simulink model "Robot"  (R2018a)
settings: Solver=VariableStepAuto  StartTime=0.0  StopTime=inf  FixedStep=1e-4  RelTol=1e-3  EnableMultiTasking=on
values from neighbouring files (symbols this model uses):
  CM730_acc_center = (4 * 9.80665)    (= 39.2266)    [CM730.m]
  CM730_acc_gain = 512 / CM730_acc_center    (= 13.0523675261)    [CM730.m]
  CM730_gyro_center = (1600 / 360 * 2 * pi)    (= 27.9252680319)    [CM730.m]
  CM730_gyro_gain = 512 / CM730_gyro_center    (= 18.3346494442)    [CM730.m]
  CM730_sample_time = 1e-3    (= 0.001)    [CM730.m]
  FSR_max = 254    [FSR.m]
  FSR_no_load = 255    [FSR.m]
  FSR_sample_time = 0.001    [FSR.m]
  FSR_scale = 1000    [FSR.m]
  g = 0    [Euler.m]
  MX106_Te = 1/1000    (= 0.001)    [MX106_init.m]
  MX28_inertia = 9e-8 * MX28_reduction^2    (= 0.0033385284)    [MX28_init.m]
  MX28_Te = 1/1000    (= 0.001)    [MX28_init.m]
  posZero_ID1 = posZero(1)    [Robot_init.m]
  posZero_ID10 = posZero(14)    [Robot_init.m]
  posZero_ID11 = posZero(9)    [Robot_init.m]
  posZero_ID12 = posZero(15)    [Robot_init.m]
  posZero_ID13 = posZero(10)    [Robot_init.m]
  posZero_ID14 = posZero(16)    [Robot_init.m]
  posZero_ID15 = posZero(11)    [Robot_init.m]
  posZero_ID16 = posZero(17)    [Robot_init.m]
  posZero_ID17 = posZero(12)    [Robot_init.m]
  posZero_ID18 = posZero(18)    [Robot_init.m]
  posZero_ID19 = posZero(19)    [Robot_init.m]
  posZero_ID2 = posZero(4)    [Robot_init.m]
  posZero_ID20 = posZero(20)    [Robot_init.m]
  posZero_ID3 = posZero(2)    [Robot_init.m]
  posZero_ID4 = posZero(5)    [Robot_init.m]
  posZero_ID5 = posZero(3)    [Robot_init.m]
  posZero_ID6 = posZero(6)    [Robot_init.m]
  posZero_ID7 = posZero(7)    [Robot_init.m]
  posZero_ID8 = posZero(13)    [Robot_init.m]
  posZero_ID9 = posZero(8)    [Robot_init.m]
  robot_chest_mass = 2385.0    (= 2385)    [Robot_init.m]
  robot_floor_friction_coeff = 0.6    [Robot_init.m]
  robot_floor_position_gain = -1e5    (= -100000)    [Robot_init.m]
  robot_floor_speed_gain = -1e3    (= -1000)    [Robot_init.m]
  robot_gravity = [0 0 0]    [Robot_init.m]
  robot_head_mass = 177.69    [Robot_init.m]
  robot_hip1_mass = 49.00    (= 49)    [Robot_init.m]
  robot_left_ankle_mass = 360.00    (= 360)    [Robot_init.m]
  robot_left_foot_mass = 267.00    (= 267)    [Robot_init.m]
  robot_left_forearm_mass = 248.00    (= 248)    [Robot_init.m]
  robot_left_hip2_mass = 358.00    (= 358)    [Robot_init.m]
  robot_left_lower_leg_mass = 129.00    (= 129)    [Robot_init.m]
  robot_left_shoulder_mass = 39.00    (= 39)    [Robot_init.m]
  robot_left_thigh_mass = 1263.00    (= 1263)    [Robot_init.m]
  robot_left_upper_arm_mass = 247.00    (= 247)    [Robot_init.m]
  robot_neck_mass = 90    [Robot_init.m]
  robot_right_ankle_mass = 360.00    (= 360)    [Robot_init.m]
  robot_right_foot_mass = 267.00    (= 267)    [Robot_init.m]
  robot_right_forearm_mass = 248.00    (= 248)    [Robot_init.m]
  robot_right_hip2_mass = 358.00    (= 358)    [Robot_init.m]
  robot_right_lower_leg_mass = 129.00    (= 129)    [Robot_init.m]
  robot_right_shoulder_mass = 39.00    (= 39)    [Robot_init.m]
  robot_right_thigh_mass = 263.00    (= 263)    [Robot_init.m]
  robot_right_upper_arm_mass = 247.00    (= 247)    [Robot_init.m]
  X = get(hObject,'Value')    [gui_kine.m]
  Y = get(hObject,'Value')    [gui_kine.m]
  Z = get(hObject,'Value')    [gui_kine.m]
libraries: sm_lib x167, fl_lib x128, nesl_utility x77, dspindex x1
(part 5 of 7)

== system Robot/Robot simulation/Right Arm/Right Shoulder Roll (3) ==
  Inertia : sm_lib/Body Elements/Inertia  InertiaType=Custom  Mass=1  MassUnits=g  CenterOfMass=[0 0 0]  CenterOfMassUnits=m  MomentsOfInertia=[0 0 MX28_inertia]  MomentsOfInertiaUnits=kg*m^2  ProductsOfInertia=[0 0 0]  ProductsOfInertiaUnits=kg*m^2  GraphicType=Marker  MarkerShape=Inertia  MarkerSize=20  GraphicVisPropType=SimpleVisualProperties  GraphicDiffuseColor=[0.5 0.5 0.5]  GraphicSpecularColor=[0.5 0.5 0.5 1.0]  GraphicAmbientColor=[0.15 0.15 0.15 1.0]  GraphicEmissiveColor=[0.0 0.0 0.0 1.0]  GraphicShininess=75  GraphicOpacity=1.0
  MX28 Command : DataStoreRead  DataStoreName=MX28_ID3  SampleTime=MX28_Te  DataStoreElements=MX28_ID3.CW_angle_limit#MX28_ID3.CCW_angle_limit#MX28_ID3.torque_enable#MX28_ID3.D_gain#MX28_ID3.I_gain#MX28_ID3.P_gain#MX28_ID3.goal_position#MX28_ID3.moving_speed#MX28_ID3.torque_limit
  MX28 State : DataStoreWrite  DataStoreName=MX28_ID3  DataStoreElements=MX28_ID3.present_position#MX28_ID3.present_speed#MX28_ID3.present_load#MX28_ID3.moving#MX28_ID3.pwm
  Model : ModelReference  ModelNameDialog=MX28.slx  SimulationMode=Normal  ModelReferenceVersion=1.66
  Position converter : nesl_utility/PS-Simulink Converter  PhysicalDomain=network_engine_domain  SubClassName=ps_output  LeftPortType=input  RightPortType=output  PseudoPeriodic=off  Frequencies=[]  Unit=rad  AffineConversion=off
  Revolute Joint : sm_lib/Joints/Revolute Joint  SenseConstraintForce=off  SenseConstraintForceX=off  SenseConstraintForceY=off  SenseConstraintForceZ=off  SenseConstraintTorque=off  SenseConstraintTorqueX=off  SenseConstraintTorqueY=off  SenseConstraintTorqueZ=off  SenseTotalForce=off  SenseTotalForceX=off  SenseTotalForceY=off  SenseTotalForceZ=off  SenseTotalTorque=off  SenseTotalTorqueX=off  SenseTotalTorqueY=off  SenseTotalTorqueZ=off  CompositeWrenchDir=FollowerOnBase  CompositeWrenchFrame=BaseFrame  EquilibriumPosition=0  EquilibriumPositionUnits=deg  SpringStiffness=0  SpringStiffnessUnits=N*m/deg  DampingCoefficient=MX28_lub_friction  DampingCoefficientUnits=N*m/(rad/s)  TorqueActuationMode=InputTorque  MotionActuationMode=ComputedMotion  SensePosition=on  SenseVelocity=on  SenseAcceleration=off  SenseTorqueForce=off  PositionTargetSpecify=on  PositionTargetPriority=High  PositionTargetValue=MX28_init_position  PositionTargetValueUnits=rad  VelocityTargetSpecify=on  VelocityTargetPriority=High  VelocityTargetValue=MX28_init_speed  VelocityTargetValueUnits=rad/s
  Speed converter : nesl_utility/PS-Simulink Converter  PhysicalDomain=network_engine_domain  SubClassName=ps_output  LeftPortType=input  RightPortType=output  PseudoPeriodic=off  Frequencies=[]  Unit=rad/s  AffineConversion=off
  Torque converter : nesl_utility/Simulink-PS Converter  PhysicalDomain=network_engine_domain  SubClassName=ps_input  LeftPortType=input  RightPortType=output  PseudoPeriodic=off  Frequencies=[]  NoiseDistribution=none  NoiseParameters=[]  Unit=N*m  AffineConversion=off  FilteringAndDerivatives=zero  SimscapeFilterOrder=1  InputFilterTimeConstant=0.001  UdotUserProvided=1
  Base : PMIOPort  Side=Left
  Axis : PMIOPort  Port=2  Side=Right
  wires:
  Model/4 -> MX28 State/3
  Model/2 -> MX28 State/1
  Model/5 -> MX28 State/4
  Model/3 -> MX28 State/2
  MX28 Command/3 -> Model/5
  MX28 Command/6 -> Model/8
  MX28 Command/4 -> Model/6
  MX28 Command/5 -> Model/7
  MX28 Command/7 -> Model/9
  MX28 Command/2 -> Model/4
  MX28 Command/1 -> Model/3
  Speed converter/1 -> Model/1
  Position converter/1 -> Model/2
  Model/1 -> Torque converter/1
  Model/6 -> MX28 State/5
  MX28 Command/8 -> Model/10
  MX28 Command/9 -> Model/11
  connections:
  Axis/RConn1 -- Revolute Joint/RConn1 -- Inertia/RConn1
  Revolute Joint/RConn3 -- Speed converter/LConn1
  Revolute Joint/RConn2 -- Position converter/LConn1
  Revolute Joint/LConn2 -- Torque converter/RConn1
  Revolute Joint/LConn1 -- Base/RConn1

== system Robot/Robot simulation/Right Arm/Right Upper Arm ==
  Right Arm Axis to Right Forearm Base : sm_lib/Frames and Transforms/Rigid Transform  TranslationMethod=Cartesian  TranslationStandardOffset=0  TranslationLengthUnit=mm  TranslationStandardAxis=+Z  TranslationCartesianOffset=robot_right_upper_arm_to_right_forearm_tra  TranslationROffset=0  TranslationROffsetUnits=m  TranslationZOffset=0  TranslationZOffsetUnits=m  TranslationThetaOffset=0  TranslationThetaOffsetUnits=deg  RotationMethod=RotationMatrix  RotationAngleUnits=deg  RotationStandardAxis=+Z  RotationAngle=0  RotationArbitraryAxis=[0 0 1]  FollAlignAxisA=+X  BaseAlignAxisA=-Y  FollAlignAxisB=+Z  BaseAlignAxisB=+X  RotationSequenceAxes=FollowerAxes  RotationSequence=XYX  RotationSequenceAngles=[0 0 0]  RotationSequenceAnglesUnits=deg  RotationMatrix=robot_right_upper_arm_to_right_forearm_rot
  Solid : sm_lib/Body Elements/Solid  InertiaType=Custom  Mass=robot_right_upper_arm_mass  MassUnits=g  CenterOfMass=robot_right_upper_arm_to_center_mass  CenterOfMassUnits=mm  MomentsOfInertia=robot_right_upper_arm_moment_inertia  MomentsOfInertiaUnits=g*mm^2  ProductsOfInertia=robot_right_upper_arm_product_inertia  ProductsOfInertiaUnits=g*mm^2  DensityBased=on  Density=1000  DensityUnits=kg/(m^3)  DoExposeReferenceFrame=on  SerializedFrames=<Frames/>  GraphicType=FromGeometry  MarkerShape=Sphere  MarkerSize=10  MarkerSizeUnits=m  GraphicVisPropType=SimpleVisualProperties  GraphicDiffuseColor=[0.5 0.5 0.5]  GraphicSpecularColor=[0.5 0.5 0.5 1.0]  GraphicAmbientColor=[0.15 0.15 0.15 1.0]  GraphicEmissiveColor=[0.0 0.0 0.0 1.0]  GraphicShininess=75  GraphicOpacity=1.0  GeometryShape=FromFile  RectangleSize=[1 1]  RectangleSizeUnits=m  BrickDimensions=[1 1 1]  BrickDimensionUnits=mm  CylinderRadius=1  CylinderRadiusUnits=m  CylinderLength=1  CylinderLengthUnits=m  SphereRadius=1  SphereRadiusUnits=m  EllipsoidRadii=[1 1 1]  EllipsoidRadiiUnits=m  ExtrusionCrossSection=[1 1; -1 1; -1 -1; 1 -1]  ExtrusionCrossSectionUnits=m  ExtrusionLength=1  ExtrusionLengthUnits=m  PolygonNumSides=3  PolygonOuterRadius=1  PolygonOuterRadiusUnits=m  ExtGeomFileType=STL  ExtGeomFileName=\STL\Right_Arm.STL  ExtGeomFileUnits=mm  RevolutionCrossSection=[1 1; 1 -1; 2 -1; 2 1]  RevolutionCrossSectionUnits=m  RevolutionExtent=Full  RevolutionAngle=180  RevolutionAngleUnits=deg
  Right Shoulder Roll : PMIOPort  Side=Left
  Right Elbow : PMIOPort  Port=2  Side=Right
  connections:
  Right Arm Axis to Right Forearm Base/LConn1 -- Right Shoulder Roll/RConn1 -- Solid/RConn1
  Right Arm Axis to Right Forearm Base/RConn1 -- Right Elbow/RConn1

== system Robot/Robot simulation/Right Leg/Floor model ==
  note: Left foot:
      | 1 = back right
      | 2 = back left
      | 3 = front left
      | 4 = front right
  note: Right foot:
      | 1 = front left
      | 2 = front right
      | 3 = back right
      | 4 = back left
  Back Left Scale : Gain  Gain=FSR_scale  OutDataTypeStr=uint16  SampleTime=FSR_sample_time  SaturateOnIntegerOverflow=on
  Back Right Scale : Gain  Gain=FSR_scale  OutDataTypeStr=uint16  SampleTime=FSR_sample_time  SaturateOnIntegerOverflow=on
  Data Store Write : DataStoreWrite  DataStoreName=FSR_ID111  DataStoreElements=FSR_ID111.fsr_1#FSR_ID111.fsr_2#FSR_ID111.fsr_3#FSR_ID111.fsr_4#FSR_ID111.fsr_x#FSR_ID111.fsr_y
  Divide X : Product  Inputs=*/
  Divide Y : Product  Inputs=*/
  Floor Model Back Left : Subsystem
  Floor Model Back Right : Subsystem
  Floor Model Front Left : Subsystem
  Floor Model Front Right : Subsystem
  Front Left Scale : Gain  Gain=FSR_scale  OutDataTypeStr=uint16  SampleTime=FSR_sample_time  SaturateOnIntegerOverflow=on
  Front Right Scale : Gain  Gain=FSR_scale  OutDataTypeStr=uint16  SampleTime=FSR_sample_time  SaturateOnIntegerOverflow=on
  Gain X : Gain  Gain=FSR_max  OutDataTypeStr=uint8  SaturateOnIntegerOverflow=on
  Gain Y : Gain  Gain=FSR_max  OutDataTypeStr=uint8  SaturateOnIntegerOverflow=on
  No load : Constant  Value=FSR_no_load  OutDataTypeStr=uint8
  Switch X : Switch  Criteria=u2 > Threshold
  Switch Y : Switch  Criteria=u2 > Threshold
  Total : Sum  Inputs=++++  SampleTime=FSR_sample_time
  Total Back : Sum  SampleTime=FSR_sample_time
  Total Right : Sum  SampleTime=FSR_sample_time
  Front Left : PMIOPort  Side=Left
  Front Right : PMIOPort  Port=2  Side=Left
  Back Right : PMIOPort  Port=3  Side=Left
  Back Left : PMIOPort  Port=4  Side=Left
  Floor : PMIOPort  Port=5  Side=Right
  wires:
  Floor Model Front Left/1(Z force) -> Total/1, Front Left Scale/1
  Floor Model Front Right/1(Z force) -> Total Right/1, Front Right Scale/1, Total/2
  Floor Model Back Right/1(Z force) -> Total Back/1, Total/3, Back Right Scale/1, Total Right/2
  Floor Model Back Left/1(Z force) -> Total Back/2, Total/4, Back Left Scale/1
  Total/1 -> Divide Y/2, Divide X/2, Switch Y/2, Switch X/2
  No load/1 -> Switch Y/3, Switch X/3
  Divide X/1 -> Gain X/1
  Total Right/1 -> Divide X/1
  Divide Y/1 -> Gain Y/1
  Total Back/1 -> Divide Y/1
  Gain X/1 -> Switch X/1
  Gain Y/1 -> Switch Y/1
  Switch X/1 -> Data Store Write/5
  Switch Y/1 -> Data Store Write/6
  Front Left Scale/1 -> Data Store Write/1
  Front Right Scale/1 -> Data Store Write/2
  Back Right Scale/1 -> Data Store Write/3
  Back Left Scale/1 -> Data Store Write/4
  connections:
  Floor Model Back Left/LConn1 -- Back Left/RConn1
  Floor Model Back Right/LConn1 -- Back Right/RConn1
  Floor Model Front Right/LConn1 -- Front Right/RConn1
  Floor Model Front Left/LConn1 -- Front Left/RConn1
  Floor/RConn1 -- Floor Model Front Left/RConn1 -- Floor Model Front Right/RConn1 -- Floor Model Back Right/RConn1 -- Floor Model Back Left/RConn1

== system Robot/Robot simulation/Right Leg/Right Ankle ==
  Right Ankle Base to Right Foot Base : sm_lib/Frames and Transforms/Rigid Transform  TranslationMethod=Cartesian  TranslationStandardOffset=0  TranslationLengthUnit=mm  TranslationStandardAxis=+Z  TranslationCartesianOffset=robot_right_ankle_to_right_foot_tra  TranslationROffset=0  TranslationROffsetUnits=m  TranslationZOffset=0  TranslationZOffsetUnits=m  TranslationThetaOffset=0  TranslationThetaOffsetUnits=deg  RotationMethod=RotationMatrix  RotationAngleUnits=deg  RotationStandardAxis=+Z  RotationAngle=0  RotationArbitraryAxis=[0 0 1]  FollAlignAxisA=+X  BaseAlignAxisA=+Z  FollAlignAxisB=+Y  BaseAlignAxisB=-Y  RotationSequenceAxes=FollowerAxes  RotationSequence=XYX  RotationSequenceAngles=[0 0 0]  RotationSequenceAnglesUnits=deg  RotationMatrix=robot_right_ankle_to_right_foot_rot
  Solid : sm_lib/Body Elements/Solid  InertiaType=Custom  Mass=robot_right_ankle_mass  MassUnits=g  CenterOfMass=robot_right_ankle_to_center_mass  CenterOfMassUnits=mm  MomentsOfInertia=robot_right_ankle_moment_inertia  MomentsOfInertiaUnits=g*mm^2  ProductsOfInertia=robot_right_ankle_product_inertia  ProductsOfInertiaUnits=g*mm^2  DensityBased=on  Density=1000  DensityUnits=kg/(m^3)  DoExposeReferenceFrame=on  SerializedFrames=<Frames/>  GraphicType=FromGeometry  MarkerShape=Sphere  MarkerSize=10  MarkerSizeUnits=m  GraphicVisPropType=SimpleVisualProperties  GraphicDiffuseColor=[0.5 0.5 0.5]  GraphicSpecularColor=[0.5 0.5 0.5 1.0]  GraphicAmbientColor=[0.15 0.15 0.15 1.0]  GraphicEmissiveColor=[0.0 0.0 0.0 1.0]  GraphicShininess=75  GraphicOpacity=1.0  GeometryShape=FromFile  RectangleSize=[1 1]  RectangleSizeUnits=m  BrickDimensions=[1 1 1]  BrickDimensionUnits=m  CylinderRadius=1  CylinderRadiusUnits=m  CylinderLength=1  CylinderLengthUnits=m  SphereRadius=1  SphereRadiusUnits=m  EllipsoidRadii=[1 1 1]  EllipsoidRadiiUnits=m  ExtrusionCrossSection=[1 1; -1 1; -1 -1; 1 -1]  ExtrusionCrossSectionUnits=m  ExtrusionLength=1  ExtrusionLengthUnits=m  PolygonNumSides=3  PolygonOuterRadius=1  PolygonOuterRadiusUnits=m  ExtGeomFileType=STL  ExtGeomFileName=\STL\Right_Ankle.STL  ExtGeomFileUnits=mm  RevolutionCrossSection=[1 1; 1 -1; 2 -1; 2 1]  RevolutionCrossSectionUnits=m  RevolutionExtent=Full  RevolutionAngle=180  RevolutionAngleUnits=deg
  Right Ankle Pitch : PMIOPort  Side=Left
  Right Ankle Roll : PMIOPort  Port=2  Side=Right
  connections:
  Solid/RConn1 -- Right Ankle Base to Right Foot Base/LConn1 -- Right Ankle Pitch/RConn1
  Right Ankle Roll/RConn1 -- Right Ankle Base to Right Foot Base/RConn1

== system Robot/Robot simulation/Right Leg/Right Ankle Pitch (15) ==
  Inertia : sm_lib/Body Elements/Inertia  InertiaType=Custom  Mass=1  MassUnits=g  CenterOfMass=[0 0 0]  CenterOfMassUnits=m  MomentsOfInertia=[0 0 MX28_inertia]  MomentsOfInertiaUnits=kg*m^2  ProductsOfInertia=[0 0 0]  ProductsOfInertiaUnits=kg*m^2  GraphicType=Marker  MarkerShape=Inertia  MarkerSize=20  GraphicVisPropType=SimpleVisualProperties  GraphicDiffuseColor=[0.5 0.5 0.5]  GraphicSpecularColor=[0.5 0.5 0.5 1.0]  GraphicAmbientColor=[0.15 0.15 0.15 1.0]  GraphicEmissiveColor=[0.0 0.0 0.0 1.0]  GraphicShininess=75  GraphicOpacity=1.0
  MX106 Command : DataStoreRead  DataStoreName=MX106_ID15  SampleTime=MX106_Te  DataStoreElements=MX106_ID15.CW_angle_limit#MX106_ID15.CCW_angle_limit#MX106_ID15.torque_enable#MX106_ID15.D_gain#MX106_ID15.I_gain#MX106_ID15.P_gain#MX106_ID15.goal_position#MX106_ID15.moving_speed#MX106_ID15.torque_limit
  MX106 State : DataStoreWrite  DataStoreName=MX106_ID15  DataStoreElements=MX106_ID15.present_position#MX106_ID15.present_speed#MX106_ID15.present_load#MX106_ID15.moving#MX106_ID15.pwm
  Model : ModelReference  ModelNameDialog=MX106.slx  SimulationMode=Normal  ModelReferenceVersion=1.67
  Position converter : nesl_utility/PS-Simulink Converter  PhysicalDomain=network_engine_domain  SubClassName=ps_output  LeftPortType=input  RightPortType=output  PseudoPeriodic=off  Frequencies=[]  Unit=rad  AffineConversion=off
  Revolute Joint : sm_lib/Joints/Revolute Joint  SenseConstraintForce=off  SenseConstraintForceX=off  SenseConstraintForceY=off  SenseConstraintForceZ=off  SenseConstraintTorque=off  SenseConstraintTorqueX=off  SenseConstraintTorqueY=off  SenseConstraintTorqueZ=off  SenseTotalForce=off  SenseTotalForceX=off  SenseTotalForceY=off  SenseTotalForceZ=off  SenseTotalTorque=off  SenseTotalTorqueX=off  SenseTotalTorqueY=off  SenseTotalTorqueZ=off  CompositeWrenchDir=FollowerOnBase  CompositeWrenchFrame=BaseFrame  EquilibriumPosition=0  EquilibriumPositionUnits=deg  SpringStiffness=0  SpringStiffnessUnits=N*m/deg  DampingCoefficient=MX28_lub_friction  DampingCoefficientUnits=N*m/(rad/s)  TorqueActuationMode=InputTorque  MotionActuationMode=ComputedMotion  SensePosition=on  SenseVelocity=on  SenseAcceleration=off  SenseTorqueForce=off  PositionTargetSpecify=on  PositionTargetPriority=High  PositionTargetValue=MX28_init_position  PositionTargetValueUnits=rad  VelocityTargetSpecify=on  VelocityTargetPriority=High  VelocityTargetValue=MX28_init_speed  VelocityTargetValueUnits=rad/s
  Speed converter : nesl_utility/PS-Simulink Converter  PhysicalDomain=network_engine_domain  SubClassName=ps_output  LeftPortType=input  RightPortType=output  PseudoPeriodic=off  Frequencies=[]  Unit=rad/s  AffineConversion=off
  Torque converter : nesl_utility/Simulink-PS Converter  PhysicalDomain=network_engine_domain  SubClassName=ps_input  LeftPortType=input  RightPortType=output  PseudoPeriodic=off  Frequencies=[]  NoiseDistribution=none  NoiseParameters=[]  Unit=N*m  AffineConversion=off  FilteringAndDerivatives=zero  SimscapeFilterOrder=1  InputFilterTimeConstant=0.001  UdotUserProvided=1
  Base : PMIOPort  Side=Left
  Axis : PMIOPort  Port=2  Side=Right
  wires:
  Model/4 -> MX106 State/3
  Model/2 -> MX106 State/1
  Model/5 -> MX106 State/4
  Model/3 -> MX106 State/2
  MX106 Command/3 -> Model/5
  MX106 Command/6 -> Model/8
  MX106 Command/4 -> Model/6
  MX106 Command/5 -> Model/7
  MX106 Command/7 -> Model/9
  MX106 Command/2 -> Model/4
  MX106 Command/1 -> Model/3
  Position converter/1 -> Model/2
  Speed converter/1 -> Model/1
  Model/1 -> Torque converter/1
  Model/6 -> MX106 State/5
  MX106 Command/8 -> Model/10
  MX106 Command/9 -> Model/11
  connections:
  Axis/RConn1 -- Revolute Joint/RConn1 -- Inertia/RConn1
  Revolute Joint/LConn1 -- Base/RConn1
  Revolute Joint/RConn3 -- Speed converter/LConn1
  Revolute Joint/RConn2 -- Position converter/LConn1
  Revolute Joint/LConn2 -- Torque converter/RConn1

== system Robot/Robot simulation/Right Leg/Right Ankle Roll (17) ==
  Inertia : sm_lib/Body Elements/Inertia  InertiaType=Custom  Mass=1  MassUnits=g  CenterOfMass=[0 0 0]  CenterOfMassUnits=m  MomentsOfInertia=[0 0 MX28_inertia]  MomentsOfInertiaUnits=kg*m^2  ProductsOfInertia=[0 0 0]  ProductsOfInertiaUnits=kg*m^2  GraphicType=Marker  MarkerShape=Inertia  MarkerSize=20  GraphicVisPropType=SimpleVisualProperties  GraphicDiffuseColor=[0.5 0.5 0.5]  GraphicSpecularColor=[0.5 0.5 0.5 1.0]  GraphicAmbientColor=[0.15 0.15 0.15 1.0]  GraphicEmissiveColor=[0.0 0.0 0.0 1.0]  GraphicShininess=75  GraphicOpacity=1.0
  MX106 Command : DataStoreRead  DataStoreName=MX106_ID17  SampleTime=MX106_Te  DataStoreElements=MX106_ID17.CW_angle_limit#MX106_ID17.CCW_angle_limit#MX106_ID17.torque_enable#MX106_ID17.D_gain#MX106_ID17.I_gain#MX106_ID17.P_gain#MX106_ID17.goal_position#MX106_ID17.moving_speed#MX106_ID17.torque_limit
  MX106 State : DataStoreWrite  DataStoreName=MX106_ID17  DataStoreElements=MX106_ID17.present_position#MX106_ID17.present_speed#MX106_ID17.present_load#MX106_ID17.moving#MX106_ID17.pwm
  Model : ModelReference  ModelNameDialog=MX106.slx  SimulationMode=Normal  ModelReferenceVersion=1.67
  Position converter : nesl_utility/PS-Simulink Converter  PhysicalDomain=network_engine_domain  SubClassName=ps_output  LeftPortType=input  RightPortType=output  PseudoPeriodic=off  Frequencies=[]  Unit=rad  AffineConversion=off
  Revolute Joint : sm_lib/Joints/Revolute Joint  SenseConstraintForce=off  SenseConstraintForceX=off  SenseConstraintForceY=off  SenseConstraintForceZ=off  SenseConstraintTorque=off  SenseConstraintTorqueX=off  SenseConstraintTorqueY=off  SenseConstraintTorqueZ=off  SenseTotalForce=off  SenseTotalForceX=off  SenseTotalForceY=off  SenseTotalForceZ=off  SenseTotalTorque=off  SenseTotalTorqueX=off  SenseTotalTorqueY=off  SenseTotalTorqueZ=off  CompositeWrenchDir=FollowerOnBase  CompositeWrenchFrame=BaseFrame  EquilibriumPosition=0  EquilibriumPositionUnits=deg  SpringStiffness=0  SpringStiffnessUnits=N*m/deg  DampingCoefficient=MX28_lub_friction  DampingCoefficientUnits=N*m/(rad/s)  TorqueActuationMode=InputTorque  MotionActuationMode=ComputedMotion  SensePosition=on  SenseVelocity=on  SenseAcceleration=off  SenseTorqueForce=off  PositionTargetSpecify=on  PositionTargetPriority=High  PositionTargetValue=MX28_init_position  PositionTargetValueUnits=rad  VelocityTargetSpecify=on  VelocityTargetPriority=High  VelocityTargetValue=MX28_init_speed  VelocityTargetValueUnits=rad/s
  Speed converter : nesl_utility/PS-Simulink Converter  PhysicalDomain=network_engine_domain  SubClassName=ps_output  LeftPortType=input  RightPortType=output  PseudoPeriodic=off  Frequencies=[]  Unit=rad/s  AffineConversion=off
  Torque converter : nesl_utility/Simulink-PS Converter  PhysicalDomain=network_engine_domain  SubClassName=ps_input  LeftPortType=input  RightPortType=output  PseudoPeriodic=off  Frequencies=[]  NoiseDistribution=none  NoiseParameters=[]  Unit=N*m  AffineConversion=off  FilteringAndDerivatives=zero  SimscapeFilterOrder=1  InputFilterTimeConstant=0.001  UdotUserProvided=1
  Base : PMIOPort  Side=Left
  Axis : PMIOPort  Port=2  Side=Right
  wires:
  Model/4 -> MX106 State/3
  Model/2 -> MX106 State/1
  Model/5 -> MX106 State/4
  Model/3 -> MX106 State/2
  MX106 Command/3 -> Model/5
  MX106 Command/6 -> Model/8
  MX106 Command/4 -> Model/6
  MX106 Command/5 -> Model/7
  MX106 Command/7 -> Model/9
  MX106 Command/2 -> Model/4
  MX106 Command/1 -> Model/3
  Position converter/1 -> Model/2
  Speed converter/1 -> Model/1
  Model/1 -> Torque converter/1
  Model/6 -> MX106 State/5
  MX106 Command/8 -> Model/10
  MX106 Command/9 -> Model/11
  connections:
  Axis/RConn1 -- Revolute Joint/RConn1 -- Inertia/RConn1
  Revolute Joint/LConn1 -- Base/RConn1
  Revolute Joint/RConn3 -- Speed converter/LConn1
  Revolute Joint/RConn2 -- Position converter/LConn1
  Revolute Joint/LConn2 -- Torque converter/RConn1

== system Robot/Robot simulation/Right Leg/Right Foot ==
  Right Foot Axis to Back Left : sm_lib/Frames and Transforms/Rigid Transform  TranslationMethod=Cartesian  TranslationStandardOffset=0  TranslationLengthUnit=mm  TranslationStandardAxis=+Z  TranslationCartesianOffset=robot_right_foot_to_back_left_floor_tra  TranslationROffset=0  TranslationROffsetUnits=m  TranslationZOffset=0  TranslationZOffsetUnits=m  TranslationThetaOffset=0  TranslationThetaOffsetUnits=deg  RotationMethod=RotationMatrix  RotationAngleUnits=deg  RotationStandardAxis=+Z  RotationAngle=0.0  RotationArbitraryAxis=[0 0 1]  FollAlignAxisA=+X  BaseAlignAxisA=-X  FollAlignAxisB=+Z  BaseAlignAxisB=-Y  RotationSequenceAxes=FollowerAxes  RotationSequence=XYX  RotationSequenceAngles=[0 0 0]  RotationSequenceAnglesUnits=deg  RotationMatrix=robot_right_foot_to_floor_rot
  Right Foot Axis to Back Right : sm_lib/Frames and Transforms/Rigid Transform  TranslationMethod=Cartesian  TranslationStandardOffset=0  TranslationLengthUnit=mm  TranslationStandardAxis=+Z  TranslationCartesianOffset=robot_right_foot_to_back_right_floor_tra  TranslationROffset=0  TranslationROffsetUnits=m  TranslationZOffset=0  TranslationZOffsetUnits=m  TranslationThetaOffset=0  TranslationThetaOffsetUnits=deg  RotationMethod=RotationMatrix  RotationAngleUnits=deg  RotationStandardAxis=+Z  RotationAngle=0.0  RotationArbitraryAxis=[0 0 1]  FollAlignAxisA=+X  BaseAlignAxisA=-X  FollAlignAxisB=+Z  BaseAlignAxisB=-Y  RotationSequenceAxes=FollowerAxes  RotationSequence=XYX  RotationSequenceAngles=[0 0 0]  RotationSequenceAnglesUnits=deg  RotationMatrix=robot_right_foot_to_floor_rot
  Right Foot Axis to Front Left : sm_lib/Frames and Transforms/Rigid Transform  TranslationMethod=Cartesian  TranslationStandardOffset=0  TranslationLengthUnit=mm  TranslationStandardAxis=+Z  TranslationCartesianOffset=robot_right_foot_to_front_left_floor_tra  TranslationROffset=0  TranslationROffsetUnits=m  TranslationZOffset=0  TranslationZOffsetUnits=m  TranslationThetaOffset=0  TranslationThetaOffsetUnits=deg  RotationMethod=RotationMatrix  RotationAngleUnits=deg  RotationStandardAxis=+Z  RotationAngle=0.0  RotationArbitraryAxis=[0 0 1]  FollAlignAxisA=+X  BaseAlignAxisA=-X  FollAlignAxisB=+Z  BaseAlignAxisB=-Y  RotationSequenceAxes=FollowerAxes  RotationSequence=XYX  RotationSequenceAngles=[0 0 0]  RotationSequenceAnglesUnits=deg  RotationMatrix=robot_right_foot_to_floor_rot
  Right Foot Axis to Front Right : sm_lib/Frames and Transforms/Rigid Transform  TranslationMethod=Cartesian  TranslationStandardOffset=0  TranslationLengthUnit=mm  TranslationStandardAxis=+Z  TranslationCartesianOffset=robot_right_foot_to_front_right_floor_tra  TranslationROffset=0  TranslationROffsetUnits=m  TranslationZOffset=0  TranslationZOffsetUnits=m  TranslationThetaOffset=0  TranslationThetaOffsetUnits=deg  RotationMethod=RotationMatrix  RotationAngleUnits=deg  RotationStandardAxis=+Z  RotationAngle=0.0  RotationArbitraryAxis=[0 0 1]  FollAlignAxisA=+X  BaseAlignAxisA=-X  FollAlignAxisB=+Z  BaseAlignAxisB=-Y  RotationSequenceAxes=FollowerAxes  RotationSequence=XYX  RotationSequenceAngles=[0 0 0]  RotationSequenceAnglesUnits=deg  RotationMatrix=robot_right_foot_to_floor_rot
  Right Foot Endefector : sm_lib/Frames and Transforms/Rigid Transform  TranslationMethod=Cartesian  TranslationStandardOffset=0  TranslationLengthUnit=mm  TranslationStandardAxis=+Z  TranslationCartesianOffset=robot_right_foot_Endefector_tra  TranslationROffset=0  TranslationROffsetUnits=m  TranslationZOffset=0  TranslationZOffsetUnits=m  TranslationThetaOffset=0  TranslationThetaOffsetUnits=deg  RotationMethod=RotationMatrix  RotationAngleUnits=deg  RotationStandardAxis=+Z  RotationAngle=0.0  RotationArbitraryAxis=[0 0 1]  FollAlignAxisA=+X  BaseAlignAxisA=-X  FollAlignAxisB=+Z  BaseAlignAxisB=-Y  RotationSequenceAxes=FollowerAxes  RotationSequence=XYX  RotationSequenceAngles=[0 0 0]  RotationSequenceAnglesUnits=deg  RotationMatrix=robot_right_foot_Endefector_rot
  Solid : sm_lib/Body Elements/Solid  InertiaType=Custom  Mass=robot_right_foot_mass  MassUnits=g  CenterOfMass=robot_right_foot_to_center_mass  CenterOfMassUnits=mm  MomentsOfInertia=robot_right_foot_moment_inertia  MomentsOfInertiaUnits=g*mm^2  ProductsOfInertia=robot_right_foot_product_inertia  ProductsOfInertiaUnits=g*mm^2  DensityBased=on  Density=1000  DensityUnits=kg/(m^3)  DoExposeReferenceFrame=on  SerializedFrames=<Frames/>  GraphicType=FromGeometry  MarkerShape=Sphere  MarkerSize=10  MarkerSizeUnits=m  GraphicVisPropType=SimpleVisualProperties  GraphicDiffuseColor=[0.5 0.5 0.5]  GraphicSpecularColor=[0.5 0.5 0.5 1.0]  GraphicAmbientColor=[0.15 0.15 0.15 1.0]  GraphicEmissiveColor=[0.0 0.0 0.0 1.0]  GraphicShininess=75  GraphicOpacity=1.0  GeometryShape=FromFile  RectangleSize=[1 1]  RectangleSizeUnits=m  BrickDimensions=[1 1 1]  BrickDimensionUnits=m  CylinderRadius=1  CylinderRadiusUnits=m  CylinderLength=1  CylinderLengthUnits=m  SphereRadius=1  SphereRadiusUnits=m  EllipsoidRadii=[1 1 1]  EllipsoidRadiiUnits=m  ExtrusionCrossSection=[1 1; -1 1; -1 -1; 1 -1]  ExtrusionCrossSectionUnits=m  ExtrusionLength=1  ExtrusionLengthUnits=m  PolygonNumSides=3  PolygonOuterRadius=1  PolygonOuterRadiusUnits=m  ExtGeomFileType=STL  ExtGeomFileName=\STL\Right_Foot.STL  ExtGeomFileUnits=mm  RevolutionCrossSection=[1 1; 1 -1; 2 -1; 2 1]  RevolutionCrossSectionUnits=m  RevolutionExtent=Full  RevolutionAngle=180  RevolutionAngleUnits=deg
  Right Ankle Roll : PMIOPort  Side=Left
  Front Left : PMIOPort  Port=2  Side=Right
  Front Right : PMIOPort  Port=3  Side=Right
  Back Right : PMIOPort  Port=4  Side=Right
  Back Left : PMIOPort  Port=5  Side=Right
  EndEfector : PMIOPort  Port=6  Side=Right
  connections:
  Right Foot Axis to Front Left/LConn1 -- Right Foot Endefector/LConn1 -- Right Foot Axis to Back Right/LConn1 -- Solid/RConn1 -- Right Ankle Roll/RConn1 -- Right Foot Axis to Back Left/LConn1 -- Right Foot Axis to Front Right/LConn1
  Front Left/RConn1 -- Right Foot Axis to Front Left/RConn1
  Back Right/RConn1 -- Right Foot Axis to Back Right/RConn1
  Front Right/RConn1 -- Right Foot Axis to Front Right/RConn1
  Back Left/RConn1 -- Right Foot Axis to Back Left/RConn1
  EndEfector/RConn1 -- Right Foot Endefector/RConn1

== system Robot/Robot simulation/Right Leg/Right Hip Pitch (11) ==
  Inertia : sm_lib/Body Elements/Inertia  InertiaType=Custom  Mass=1  MassUnits=g  CenterOfMass=[0 0 0]  CenterOfMassUnits=m  MomentsOfInertia=[0 0 MX28_inertia]  MomentsOfInertiaUnits=kg*m^2  ProductsOfInertia=[0 0 0]  ProductsOfInertiaUnits=kg*m^2  GraphicType=Marker  MarkerShape=Inertia  MarkerSize=20  GraphicVisPropType=SimpleVisualProperties  GraphicDiffuseColor=[0.5 0.5 0.5]  GraphicSpecularColor=[0.5 0.5 0.5 1.0]  GraphicAmbientColor=[0.15 0.15 0.15 1.0]  GraphicEmissiveColor=[0.0 0.0 0.0 1.0]  GraphicShininess=75  GraphicOpacity=1.0
  MX106 Command : DataStoreRead  DataStoreName=MX106_ID11  SampleTime=MX106_Te  DataStoreElements=MX106_ID11.CW_angle_limit#MX106_ID11.CCW_angle_limit#MX106_ID11.torque_enable#MX106_ID11.D_gain#MX106_ID11.I_gain#MX106_ID11.P_gain#MX106_ID11.goal_position#MX106_ID11.moving_speed#MX106_ID11.torque_limit
  MX106 State : DataStoreWrite  DataStoreName=MX106_ID11  DataStoreElements=MX106_ID11.present_position#MX106_ID11.present_speed#MX106_ID11.present_load#MX106_ID11.moving#MX106_ID11.pwm
  Model : ModelReference  ModelNameDialog=MX106.slx  SimulationMode=Normal  ModelReferenceVersion=1.67
  Position converter : nesl_utility/PS-Simulink Converter  PhysicalDomain=network_engine_domain  SubClassName=ps_output  LeftPortType=input  RightPortType=output  PseudoPeriodic=off  Frequencies=[]  Unit=rad  AffineConversion=off
  Revolute Joint : sm_lib/Joints/Revolute Joint  SenseConstraintForce=off  SenseConstraintForceX=off  SenseConstraintForceY=off  SenseConstraintForceZ=off  SenseConstraintTorque=off  SenseConstraintTorqueX=off  SenseConstraintTorqueY=off  SenseConstraintTorqueZ=off  SenseTotalForce=off  SenseTotalForceX=off  SenseTotalForceY=off  SenseTotalForceZ=off  SenseTotalTorque=off  SenseTotalTorqueX=off  SenseTotalTorqueY=off  SenseTotalTorqueZ=off  CompositeWrenchDir=FollowerOnBase  CompositeWrenchFrame=BaseFrame  EquilibriumPosition=0  EquilibriumPositionUnits=deg  SpringStiffness=0  SpringStiffnessUnits=N*m/deg  DampingCoefficient=MX28_lub_friction  DampingCoefficientUnits=N*m/(rad/s)  TorqueActuationMode=InputTorque  MotionActuationMode=ComputedMotion  SensePosition=on  SenseVelocity=on  SenseAcceleration=off  SenseTorqueForce=off  PositionTargetSpecify=on  PositionTargetPriority=High  PositionTargetValue=MX28_init_position  PositionTargetValueUnits=rad  VelocityTargetSpecify=on  VelocityTargetPriority=High  VelocityTargetValue=MX28_init_speed  VelocityTargetValueUnits=rad/s
  Speed converter : nesl_utility/PS-Simulink Converter  PhysicalDomain=network_engine_domain  SubClassName=ps_output  LeftPortType=input  RightPortType=output  PseudoPeriodic=off  Frequencies=[]  Unit=rad/s  AffineConversion=off
  Torque converter : nesl_utility/Simulink-PS Converter  PhysicalDomain=network_engine_domain  SubClassName=ps_input  LeftPortType=input  RightPortType=output  PseudoPeriodic=off  Frequencies=[]  NoiseDistribution=none  NoiseParameters=[]  Unit=N*m  AffineConversion=off  FilteringAndDerivatives=zero  SimscapeFilterOrder=1  InputFilterTimeConstant=0.001  UdotUserProvided=1
  Base : PMIOPort  Side=Left
  Axis : PMIOPort  Port=2  Side=Right
  wires:
  Model/4 -> MX106 State/3
  Model/2 -> MX106 State/1
  Model/5 -> MX106 State/4
  Model/3 -> MX106 State/2
  MX106 Command/3 -> Model/5
  MX106 Command/6 -> Model/8
  MX106 Command/4 -> Model/6
  MX106 Command/5 -> Model/7
  MX106 Command/7 -> Model/9
  MX106 Command/2 -> Model/4
  MX106 Command/1 -> Model/3
  Position converter/1 -> Model/2
  Speed converter/1 -> Model/1
  Model/1 -> Torque converter/1
  Model/6 -> MX106 State/5
  MX106 Command/8 -> Model/10
  MX106 Command/9 -> Model/11
  connections:
  Axis/RConn1 -- Revolute Joint/RConn1 -- Inertia/RConn1
  Revolute Joint/LConn1 -- Base/RConn1
  Revolute Joint/RConn3 -- Speed converter/LConn1
  Revolute Joint/RConn2 -- Position converter/LConn1
  Revolute Joint/LConn2 -- Torque converter/RConn1

== system Robot/Robot simulation/Right Leg/Right Hip Roll ==
  Right Hip Roll Base to Right Hip Pitch Base : sm_lib/Frames and Transforms/Rigid Transform  TranslationMethod=Cartesian  TranslationStandardOffset=0  TranslationLengthUnit=mm  TranslationStandardAxis=+Z  TranslationCartesianOffset=robot_right_hip2_to_right_thigh_tra  TranslationROffset=0  TranslationROffsetUnits=m  TranslationZOffset=0  TranslationZOffsetUnits=m  TranslationThetaOffset=0  TranslationThetaOffsetUnits=deg  RotationMethod=RotationMatrix  RotationAngleUnits=deg  RotationStandardAxis=+Z  RotationAngle=0  RotationArbitraryAxis=[0 0 1]  FollAlignAxisA=+Z  BaseAlignAxisA=+X  FollAlignAxisB=+Y  BaseAlignAxisB=+Y  RotationSequenceAxes=FollowerAxes  RotationSequence=XYX  RotationSequenceAngles=[0 0 0]  RotationSequenceAnglesUnits=deg  RotationMatrix=robot_right_hip2_to_right_thigh_rot
  Solid : sm_lib/Body Elements/Solid  InertiaType=Custom  Mass=robot_right_hip2_mass  MassUnits=g  CenterOfMass=robot_right_hip2_to_center_mass  CenterOfMassUnits=mm  MomentsOfInertia=robot_right_hip2_moment_inertia  MomentsOfInertiaUnits=g*mm^2  ProductsOfInertia=robot_right_hip2_product_inertia  ProductsOfInertiaUnits=g*mm^2  DensityBased=on  Density=1000  DensityUnits=kg/(m^3)  DoExposeReferenceFrame=on  SerializedFrames=<Frames/>  GraphicType=FromGeometry  MarkerShape=Sphere  MarkerSize=10  MarkerSizeUnits=m  GraphicVisPropType=SimpleVisualProperties  GraphicDiffuseColor=[0.5 0.5 0.5]  GraphicSpecularColor=[0.5 0.5 0.5 1.0]  GraphicAmbientColor=[0.15 0.15 0.15 1.0]  GraphicEmissiveColor=[0.0 0.0 0.0 1.0]  GraphicShininess=75  GraphicOpacity=1.0  GeometryShape=FromFile  RectangleSize=[1 1]  RectangleSizeUnits=m  BrickDimensions=[1 1 1]  BrickDimensionUnits=mm  CylinderRadius=1  CylinderRadiusUnits=m  CylinderLength=1  CylinderLengthUnits=m  SphereRadius=1  SphereRadiusUnits=m  EllipsoidRadii=[1 1 1]  EllipsoidRadiiUnits=m  ExtrusionCrossSection=[1 1; -1 1; -1 -1; 1 -1]  ExtrusionCrossSectionUnits=m  ExtrusionLength=1  ExtrusionLengthUnits=m  PolygonNumSides=3  PolygonOuterRadius=1  PolygonOuterRadiusUnits=m  ExtGeomFileType=STL  ExtGeomFileName=\STL\Right_Hip2.STL  ExtGeomFileUnits=mm  RevolutionCrossSection=[1 1; 1 -1; 2 -1; 2 1]  RevolutionCrossSectionUnits=m  RevolutionExtent=Full  RevolutionAngle=180  RevolutionAngleUnits=deg
  Right Hip Roll : PMIOPort  Side=Left
  Right Hip Pitch : PMIOPort  Port=2  Side=Right
  connections:
  Right Hip Roll Base to Right Hip Pitch Base/LConn1 -- Solid/RConn1 -- Right Hip Roll/RConn1
  Right Hip Roll Base to Right Hip Pitch Base/RConn1 -- Right Hip Pitch/RConn1

== system Robot/Robot simulation/Right Leg/Right Hip Roll (9) ==
  Inertia : sm_lib/Body Elements/Inertia  InertiaType=Custom  Mass=1  MassUnits=g  CenterOfMass=[0 0 0]  CenterOfMassUnits=m  MomentsOfInertia=[0 0 MX28_inertia]  MomentsOfInertiaUnits=kg*m^2  ProductsOfInertia=[0 0 0]  ProductsOfInertiaUnits=kg*m^2  GraphicType=Marker  MarkerShape=Inertia  MarkerSize=20  GraphicVisPropType=SimpleVisualProperties  GraphicDiffuseColor=[0.5 0.5 0.5]  GraphicSpecularColor=[0.5 0.5 0.5 1.0]  GraphicAmbientColor=[0.15 0.15 0.15 1.0]  GraphicEmissiveColor=[0.0 0.0 0.0 1.0]  GraphicShininess=75  GraphicOpacity=1.0
  MX106 Command : DataStoreRead  DataStoreName=MX106_ID9  SampleTime=MX106_Te  DataStoreElements=MX106_ID9.CW_angle_limit#MX106_ID9.CCW_angle_limit#MX106_ID9.torque_enable#MX106_ID9.D_gain#MX106_ID9.I_gain#MX106_ID9.P_gain#MX106_ID9.goal_position#MX106_ID9.moving_speed#MX106_ID9.torque_limit
  MX106 State : DataStoreWrite  DataStoreName=MX106_ID9  DataStoreElements=MX106_ID9.present_position#MX106_ID9.present_speed#MX106_ID9.present_load#MX106_ID9.moving#MX106_ID9.pwm
  Model : ModelReference  ModelNameDialog=MX106.slx  SimulationMode=Normal  ModelReferenceVersion=1.67
  Position converter : nesl_utility/PS-Simulink Converter  PhysicalDomain=network_engine_domain  SubClassName=ps_output  LeftPortType=input  RightPortType=output  PseudoPeriodic=off  Frequencies=[]  Unit=rad  AffineConversion=off
  Revolute Joint : sm_lib/Joints/Revolute Joint  SenseConstraintForce=off  SenseConstraintForceX=off  SenseConstraintForceY=off  SenseConstraintForceZ=off  SenseConstraintTorque=off  SenseConstraintTorqueX=off  SenseConstraintTorqueY=off  SenseConstraintTorqueZ=off  SenseTotalForce=off  SenseTotalForceX=off  SenseTotalForceY=off  SenseTotalForceZ=off  SenseTotalTorque=off  SenseTotalTorqueX=off  SenseTotalTorqueY=off  SenseTotalTorqueZ=off  CompositeWrenchDir=FollowerOnBase  CompositeWrenchFrame=BaseFrame  EquilibriumPosition=0  EquilibriumPositionUnits=deg  SpringStiffness=0  SpringStiffnessUnits=N*m/deg  DampingCoefficient=MX28_lub_friction  DampingCoefficientUnits=N*m/(rad/s)  TorqueActuationMode=InputTorque  MotionActuationMode=ComputedMotion  SensePosition=on  SenseVelocity=on  SenseAcceleration=off  SenseTorqueForce=off  PositionTargetSpecify=on  PositionTargetPriority=High  PositionTargetValue=MX28_init_position  PositionTargetValueUnits=rad  VelocityTargetSpecify=on  VelocityTargetPriority=High  VelocityTargetValue=MX28_init_speed  VelocityTargetValueUnits=rad/s
  Speed converter : nesl_utility/PS-Simulink Converter  PhysicalDomain=network_engine_domain  SubClassName=ps_output  LeftPortType=input  RightPortType=output  PseudoPeriodic=off  Frequencies=[]  Unit=rad/s  AffineConversion=off
  Torque converter : nesl_utility/Simulink-PS Converter  PhysicalDomain=network_engine_domain  SubClassName=ps_input  LeftPortType=input  RightPortType=output  PseudoPeriodic=off  Frequencies=[]  NoiseDistribution=none  NoiseParameters=[]  Unit=N*m  AffineConversion=off  FilteringAndDerivatives=zero  SimscapeFilterOrder=1  InputFilterTimeConstant=0.001  UdotUserProvided=1
  Base : PMIOPort  Side=Left
  Axis : PMIOPort  Port=2  Side=Right
  wires:
  Model/4 -> MX106 State/3
  Model/2 -> MX106 State/1
  Model/5 -> MX106 State/4
  Model/3 -> MX106 State/2
  MX106 Command/3 -> Model/5
  MX106 Command/6 -> Model/8
  MX106 Command/4 -> Model/6
  MX106 Command/5 -> Model/7
  MX106 Command/7 -> Model/9
  MX106 Command/2 -> Model/4
  MX106 Command/1 -> Model/3
  Speed converter/1 -> Model/1
  Position converter/1 -> Model/2
  Model/1 -> Torque converter/1
  Model/6 -> MX106 State/5
  MX106 Command/8 -> Model/10
  MX106 Command/9 -> Model/11
  connections:
  Axis/RConn1 -- Revolute Joint/RConn1 -- Inertia/RConn1
  Revolute Joint/LConn1 -- Base/RConn1
  Revolute Joint/RConn3 -- Speed converter/LConn1
  Revolute Joint/RConn2 -- Position converter/LConn1
  Revolute Joint/LConn2 -- Torque converter/RConn1

== system Robot/Robot simulation/Right Leg/Right Hip Yaw ==
  Right Hip Yaw Axis to Right Hip Roll Axis : sm_lib/Frames and Transforms/Rigid Transform  TranslationMethod=Cartesian  TranslationStandardOffset=0  TranslationLengthUnit=mm  TranslationStandardAxis=+Z  TranslationCartesianOffset=robot_hip1_to_hip2_tra  TranslationROffset=0  TranslationROffsetUnits=m  TranslationZOffset=0  TranslationZOffsetUnits=m  TranslationThetaOffset=0  TranslationThetaOffsetUnits=deg  RotationMethod=RotationMatrix  RotationAngleUnits=deg  RotationStandardAxis=+Z  RotationAngle=0  RotationArbitraryAxis=[0 0 1]  FollAlignAxisA=+Y  BaseAlignAxisA=+Z  FollAlignAxisB=+X  BaseAlignAxisB=-Y  RotationSequenceAxes=FollowerAxes  RotationSequence=XYX  RotationSequenceAngles=[0 0 0]  RotationSequenceAnglesUnits=deg  RotationMatrix=robot_hip1_to_hip2_rot
  Solid : sm_lib/Body Elements/Solid  InertiaType=Custom  Mass=robot_hip1_mass  MassUnits=g  CenterOfMass=robot_hip1_to_center_mass  CenterOfMassUnits=mm  MomentsOfInertia=robot_hip1_moment_inertia  MomentsOfInertiaUnits=g*mm^2  ProductsOfInertia=robot_hip1_product_inertia  ProductsOfInertiaUnits=g*mm^2  DensityBased=on  Density=1000  DensityUnits=kg/(m^3)  DoExposeReferenceFrame=on  SerializedFrames=<Frames/>  GraphicType=FromGeometry  MarkerShape=Sphere  MarkerSize=10  MarkerSizeUnits=m  GraphicVisPropType=SimpleVisualProperties  GraphicDiffuseColor=[0.5 0.5 0.5]  GraphicSpecularColor=[0.5 0.5 0.5 1.0]  GraphicAmbientColor=[0.15 0.15 0.15 1.0]  GraphicEmissiveColor=[0.0 0.0 0.0 1.0]  GraphicShininess=75  GraphicOpacity=1.0  GeometryShape=FromFile  RectangleSize=[1 1]  RectangleSizeUnits=m  BrickDimensions=[1 1 1]  BrickDimensionUnits=mm  CylinderRadius=1  CylinderRadiusUnits=m  CylinderLength=1  CylinderLengthUnits=m  SphereRadius=1  SphereRadiusUnits=m  EllipsoidRadii=[1 1 1]  EllipsoidRadiiUnits=m  ExtrusionCrossSection=[1 1; -1 1; -1 -1; 1 -1]  ExtrusionCrossSectionUnits=m  ExtrusionLength=1  ExtrusionLengthUnits=m  PolygonNumSides=3  PolygonOuterRadius=1  PolygonOuterRadiusUnits=m  ExtGeomFileType=STL  ExtGeomFileName=\STL\Hip1.STL  ExtGeomFileUnits=mm  RevolutionCrossSection=[1 1; 1 -1; 2 -1; 2 1]  RevolutionCrossSectionUnits=m  RevolutionExtent=Full  RevolutionAngle=180  RevolutionAngleUnits=deg
  Right Hip Yaw : PMIOPort  Side=Left
  Right Hip Roll : PMIOPort  Port=2  Side=Right
  connections:
  Right Hip Yaw Axis to Right Hip Roll Axis/RConn1 -- Right Hip Roll/RConn1
  Solid/RConn1 -- Right Hip Yaw Axis to Right Hip Roll Axis/LConn1 -- Right Hip Yaw/RConn1

== system Robot/Robot simulation/Right Leg/Right Hip Yaw (7) ==
  Inertia : sm_lib/Body Elements/Inertia  InertiaType=Custom  Mass=1  MassUnits=g  CenterOfMass=[0 0 0]  CenterOfMassUnits=m  MomentsOfInertia=[0 0 MX28_inertia]  MomentsOfInertiaUnits=kg*m^2  ProductsOfInertia=[0 0 0]  ProductsOfInertiaUnits=kg*m^2  GraphicType=Marker  MarkerShape=Inertia  MarkerSize=20  GraphicVisPropType=SimpleVisualProperties  GraphicDiffuseColor=[0.5 0.5 0.5]  GraphicSpecularColor=[0.5 0.5 0.5 1.0]  GraphicAmbientColor=[0.15 0.15 0.15 1.0]  GraphicEmissiveColor=[0.0 0.0 0.0 1.0]  GraphicShininess=75  GraphicOpacity=1.0
  MX106 Command : DataStoreRead  DataStoreName=MX106_ID7  SampleTime=MX106_Te  DataStoreElements=MX106_ID7.CW_angle_limit#MX106_ID7.CCW_angle_limit#MX106_ID7.torque_enable#MX106_ID7.D_gain#MX106_ID7.I_gain#MX106_ID7.P_gain#MX106_ID7.goal_position#MX106_ID7.moving_speed#MX106_ID7.torque_limit
  MX106 State : DataStoreWrite  DataStoreName=MX106_ID7  DataStoreElements=MX106_ID7.present_position#MX106_ID7.present_speed#MX106_ID7.present_load#MX106_ID7.moving#MX106_ID7.pwm
  Model : ModelReference  ModelNameDialog=MX106.slx  SimulationMode=Normal  ModelReferenceVersion=1.67
  Position converter : nesl_utility/PS-Simulink Converter  PhysicalDomain=network_engine_domain  SubClassName=ps_output  LeftPortType=input  RightPortType=output  PseudoPeriodic=off  Frequencies=[]  Unit=rad  AffineConversion=off
  Revolute Joint : sm_lib/Joints/Revolute Joint  SenseConstraintForce=off  SenseConstraintForceX=off  SenseConstraintForceY=off  SenseConstraintForceZ=off  SenseConstraintTorque=off  SenseConstraintTorqueX=off  SenseConstraintTorqueY=off  SenseConstraintTorqueZ=off  SenseTotalForce=off  SenseTotalForceX=off  SenseTotalForceY=off  SenseTotalForceZ=off  SenseTotalTorque=off  SenseTotalTorqueX=off  SenseTotalTorqueY=off  SenseTotalTorqueZ=off  CompositeWrenchDir=FollowerOnBase  CompositeWrenchFrame=BaseFrame  EquilibriumPosition=0  EquilibriumPositionUnits=deg  SpringStiffness=0  SpringStiffnessUnits=N*m/deg  DampingCoefficient=MX28_lub_friction  DampingCoefficientUnits=N*m/(rad/s)  TorqueActuationMode=InputTorque  MotionActuationMode=ComputedMotion  SensePosition=on  SenseVelocity=on  SenseAcceleration=off  SenseTorqueForce=off  PositionTargetSpecify=on  PositionTargetPriority=High  PositionTargetValue=MX28_init_position  PositionTargetValueUnits=rad  VelocityTargetSpecify=on  VelocityTargetPriority=High  VelocityTargetValue=MX28_init_speed  VelocityTargetValueUnits=rad/s
  Speed converter : nesl_utility/PS-Simulink Converter  PhysicalDomain=network_engine_domain  SubClassName=ps_output  LeftPortType=input  RightPortType=output  PseudoPeriodic=off  Frequencies=[]  Unit=rad/s  AffineConversion=off
  Torque converter : nesl_utility/Simulink-PS Converter  PhysicalDomain=network_engine_domain  SubClassName=ps_input  LeftPortType=input  RightPortType=output  PseudoPeriodic=off  Frequencies=[]  NoiseDistribution=none  NoiseParameters=[]  Unit=N*m  AffineConversion=off  FilteringAndDerivatives=zero  SimscapeFilterOrder=1  InputFilterTimeConstant=0.001  UdotUserProvided=1
  Base : PMIOPort  Side=Left
  Axis : PMIOPort  Port=2  Side=Right
  wires:
  Model/4 -> MX106 State/3
  Model/2 -> MX106 State/1
  Model/5 -> MX106 State/4
  Model/3 -> MX106 State/2
  MX106 Command/3 -> Model/5
  MX106 Command/6 -> Model/8
  MX106 Command/4 -> Model/6
  MX106 Command/5 -> Model/7
  MX106 Command/7 -> Model/9
  MX106 Command/2 -> Model/4
  MX106 Command/1 -> Model/3
  Speed converter/1 -> Model/1
  Position converter/1 -> Model/2
  Model/1 -> Torque converter/1
  Model/6 -> MX106 State/5
  MX106 Command/8 -> Model/10
  MX106 Command/9 -> Model/11
  connections:
  Axis/RConn1 -- Revolute Joint/RConn1 -- Inertia/RConn1
  Revolute Joint/LConn1 -- Base/RConn1
  Revolute Joint/RConn3 -- Speed converter/LConn1
  Revolute Joint/RConn2 -- Position converter/LConn1
  Revolute Joint/LConn2 -- Torque converter/RConn1
